simulink model "A_FSK"  (Simulink 8.3)
settings: Solver=ode45  StartTime=0.0  StopTime=sim_t  RelTol=1e-3
undefined symbols (not defined in the file): A0f, A1f, BSTf, F0f, F1f, PZf, STf
libraries: commrandsrc2 x1, commsynccomp2 x1
settings Model: Creator=usuario  LastModifiedBy=Cocheka
settings OptimizationCC: ExpressionDepthLimit=2147483647  InitFltsAndDblsToZero=on
settings DebuggingCC: SaveWithParameterizedLinksMsg=none  SignalResolutionControl=TryResolveAllWithWarning  MultiTaskDSMMsg=warning  MultiTaskCondExecSysMsg=none  FcnCallInpInsideContextMsg=UseLocalSettings
settings RTWCC: IncludeERTFirstTime=on
settings GRTTargetCC: TargetFcnLib=ansi_tfl_tmw.mat

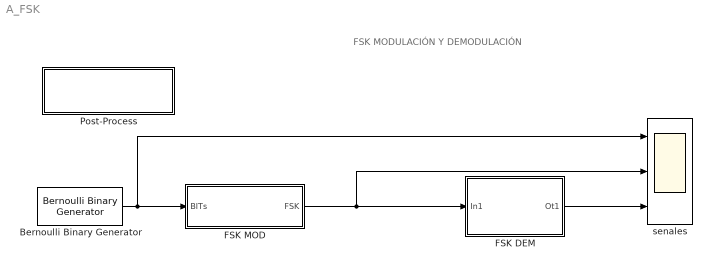
== system A_FSK ==
  note: FSK MODULACIÓN Y DEMODULACIÓN
  Bernoulli Binary Generator : commrandsrc2/Bernoulli Binary Generator  P=PZf  seed=61  Ts=BSTf  frameBased=off  sampPerFrame=1  orient=off  outDataType=double
  FSK DEM : Subsystem
  FSK MOD : Subsystem
  Post-Process : Subsystem  mask{sim_t=50, BSTf=5, F1f=6000, A1f=1, F0f=12000, A0f=1}
      mask prompts: sim_t "Sim Time [100]"; BSTf "Source Sample Time"; F1f "Freq. Sine 1 [8K]"; A1f "Amp. Sine 1 [1]"; F0f "Freq. Sine 0 [12K]"; A0f "Amp. Sine 0 [1]"
      mask init:
      | %sim_t = 100; %simulation time
      | %BSTf = 5; % source sample time
      | PZf = .3; % probability of zero
      | 
      | %STf = 1/100; % sample time
      | %A1f = 1; % amplitude sine 1 - mod.
      | %A2f = 1; % amplitude sine 2 - mod.
      | %F1f = 2*pi*8; % Freg Sine 1
      | %F2f = 2*pi*12; % Freg Sine 2
      | 
      | switch sim_t
      |     case 1
      |         sim_t = 25;
      |     case 2
      |         sim_t = 50;
      |     case 3
      |         sim_t = 100;
      |     case 4
      |         sim_t = 150;   
      | end
      | 
      | % Sample Time Source Configure
      | switch BSTf
      |     case 1
      |         BSTf = 3;
      |     case 2
      |         BSTf = 5;
      |     case 3
      |         BSTf = 8;
      |     case 4
      |         BSTf = 10;
      |     case 5
      |         BSTf = 12;        
      | end
      | 
      | switch F1f
      |     case 1
      |         F1f = 6000;
      |     case 2
      |         F1f = 8000;
      |     case 3
      |         F1f = 10000;
      |     case 4
      |         F1f = 16000;
      | end
      | 
      | switch F0f
      |     case 1
      |         F0f = 8000;
      |     case 2    
      |         F0f = 10000;
      |     case 3        
      |         F0f = 12000;
      |     case 4
      |         F0f = 16000;
      | end
      | 
      | STf=(1/BSTf*5/100);
      | F1f=2*pi*F1f/1000;
      | F0f=2*pi*F0f/1000;
      | 
      | assignin('base','sim_t', sim_t );
      | assignin('base','BSTf', BSTf );
      | assignin('base','PZf', PZf );
      | assignin('base','STf', STf );
      | assignin('base','A1f', A1f );
      | assignin('base','A0f', A0f );
      | assignin('base','F1f', F1f );
      | assignin('base','F0f', F0f );
      mask TypeOptions sim_t: 25 | 50 | 100 | 250
      mask TypeOptions BSTf: 3 | 5 | 8 | 10 | 12
      mask TypeOptions F1f: 6000 | 8000 | 10000 | 16000
      mask TypeOptions F0f: 8000 | 10000 | 12000 | 16000
      mask Display: disp('Sim Parameters')
  senales : Scope  NumInputPorts=3
      settings: YMin=-0.5~-2~-0.5  YMax=1.5~2~1.5
  wires:
  Bernoulli Binary Generator/1 -> FSK MOD/1(BITs), senales/1
  FSK MOD/1(FSK) -> FSK DEM/1(In1), senales/2
  FSK DEM/1(Ot1) -> senales/3

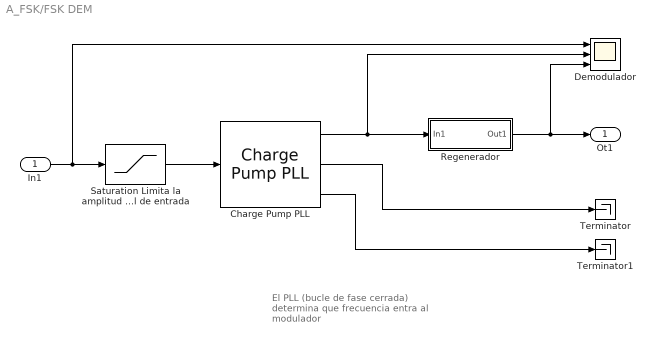
== system A_FSK/FSK DEM ==
  note: El PLL (bucle de fase cerrada)
      | determina que frecuencia
      | entra al modulador
  In1 : Inport
  Charge Pump PLL : commsynccomp2/Charge Pump PLL  Fn=[2*pi*1]  Fd="[1   2*pi*1]"  Kvco=4  Fc=10  Ph=0  Ac=1
  Demodulador : Scope  NumInputPorts=3
      settings: YMin=-2~-1~-0.5  YMax=2~1~1.5  SaveName=ScopeData2
  Regenerador : Subsystem
  Saturation Limita la amplitud de la señal de entrada : Saturate
  Terminator : Terminator
  Terminator1 : Terminator
  Ot1 : Outport
  wires:
  Saturation Limita la amplitud de la señal de entrada/1 -> Charge Pump PLL/1
  Charge Pump PLL/2 -> Terminator/1
  Charge Pump PLL/3 -> Terminator1/1
  Charge Pump PLL/1 -> Demodulador/2, Regenerador/1(In1)
  Regenerador/1(Out1) -> Demodulador/3, Ot1/1
  In1/1 -> Demodulador/1, Saturation Limita la amplitud de la señal de entrada/1

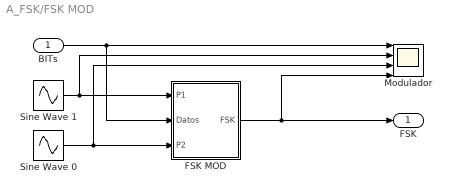
== system A_FSK/FSK MOD ==
  BITs : Inport
  FSK MOD : Subsystem
  Modulador : Scope  NumInputPorts=4
      settings: YMin=-0.5~-3~-3~-3  YMax=1.5~3~3~3
  Sine Wave 0 : Sin  Amplitude=A0f  Frequency=F0f  Samples=25  SampleTime=STf
  Sine Wave 1 : Sin  Amplitude=A1f  Frequency=F1f  Samples=50  SampleTime=STf
  FSK : Outport
  wires:
  BITs/1 -> Modulador/1, FSK MOD/2(Datos)
  FSK MOD/1(FSK) -> Modulador/4, FSK/1
  Sine Wave 1/1 -> Modulador/2, FSK MOD/1(P1)
  Sine Wave 0/1 -> Modulador/3, FSK MOD/3(P2)

== system A_FSK/Post-Process ==

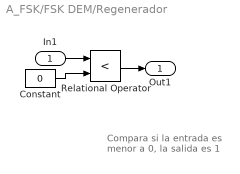
== system A_FSK/FSK DEM/Regenerador ==
  note: Compara si la entrada
      | es menor a 0, la salida es 1
  In1 : Inport
  Constant : Constant  Value=0
  Relational Operator : RelationalOperator  Operator=<  OutDataTypeStr=boolean
  Out1 : Outport
  wires:
  Relational Operator/1 -> Out1/1
  In1/1 -> Relational Operator/1
  Constant/1 -> Relational Operator/2

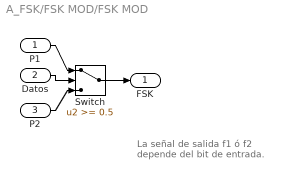
== system A_FSK/FSK MOD/FSK MOD ==
  note: La señal de salida f1 ó f2
      | depende del bit de entrada.
  P1 : Inport
  Datos : Inport  Port=2
  P2 : Inport  Port=3
  Switch : Switch  Threshold=0.5
  FSK : Outport
  wires:
  P1/1 -> Switch/1
  Datos/1 -> Switch/2
  Switch/1 -> FSK/1
  P2/1 -> Switch/3
